simulink model "elso"  (R2018a)
settings: Solver=VariableStepAuto  StartTime=0.0  StopTime=50  RelTol=1e-3
libraries: simulink x1
settings Model: Creator=alfac  LastModifiedBy=alfac

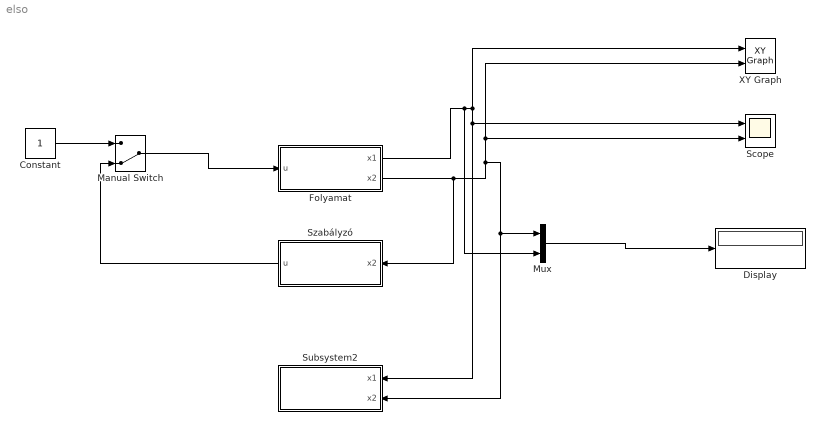
== system elso ==
  Constant : Constant
  Display : Display
  Folyamat : Subsystem  mask{omega=6, x0=[6; 10]}
  Manual Switch : ManualSwitch  CurrentSetting=0
  Mux : Mux  Inputs=2
  Scope : Scope  NumInputPorts=2
  Subsystem2 : Subsystem  mask{epszilon=0.01}
  Szabályzó : Subsystem
  XY Graph : simulink/Sinks/XY Graph  xmin=-1  xmax=1  ymin=-1  ymax=1  st=-1
  wires:
  Manual Switch/1 -> Folyamat/1(u)
  Constant/1 -> Manual Switch/1
  Folyamat/1(x1) -> Mux/2, Subsystem2/1(x1), Scope/1, XY Graph/1
  Folyamat/2(x2) -> Szabályzó/1(x2), Subsystem2/2(x2), Mux/1, XY Graph/2, Scope/2
  Szabályzó/1(u) -> Manual Switch/2
  Mux/1 -> Display/1

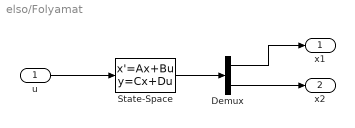
== system elso/Folyamat ==
  u : Inport
  Demux : Demux  Outputs=2
  State-Space : StateSpace  A=[0 omega; -omega 0]  B=[0; 1]  C=[1 0; 0 1]  D=[0; 0]  InitialCondition=x0
  x1 : Outport
  x2 : Outport  Port=2
  wires:
  u/1 -> State-Space/1
  State-Space/1 -> Demux/1
  Demux/1 -> x1/1
  Demux/2 -> x2/1

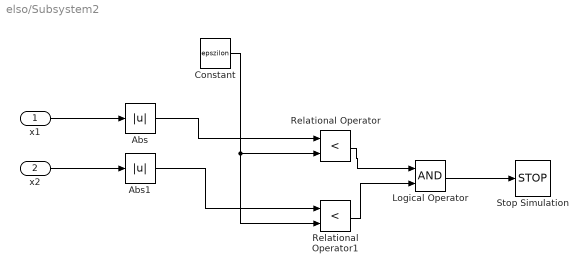
== system elso/Subsystem2 ==
  x1 : Inport
  x2 : Inport  Port=2
  Abs : Abs
  Abs1 : Abs
  Constant : Constant  Value=epszilon
  Logical Operator : Logic  AllPortsSameDT=off  OutDataTypeStr=boolean
  Relational Operator : RelationalOperator  Operator=<  OutDataTypeStr=boolean  RndMeth=Simplest
  Relational Operator1 : RelationalOperator  Operator=<  OutDataTypeStr=boolean  RndMeth=Simplest
  Stop Simulation : Stop
  wires:
  x1/1 -> Abs/1
  x2/1 -> Abs1/1
  Constant/1 -> Relational Operator1/2, Relational Operator/2
  Abs1/1 -> Relational Operator1/1
  Relational Operator/1 -> Logical Operator/1
  Relational Operator1/1 -> Logical Operator/2
  Abs/1 -> Relational Operator/1
  Logical Operator/1 -> Stop Simulation/1

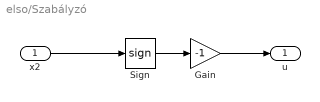
== system elso/Szabályzó ==
  x2 : Inport
  Gain : Gain  Gain=-1
  Sign : Signum
  u : Outport
  wires:
  Gain/1 -> u/1
  Sign/1 -> Gain/1
  x2/1 -> Sign/1
